simulink model "pi_controllers"  (R2018a)
settings: Solver=VariableStepAuto  StartTime=0.0  StopTime=5  RelTol=1e-3
libraries: fuzblock x1, simulink x1
settings Model: Creator=Iasonas  LastModifiedBy=Iasonas

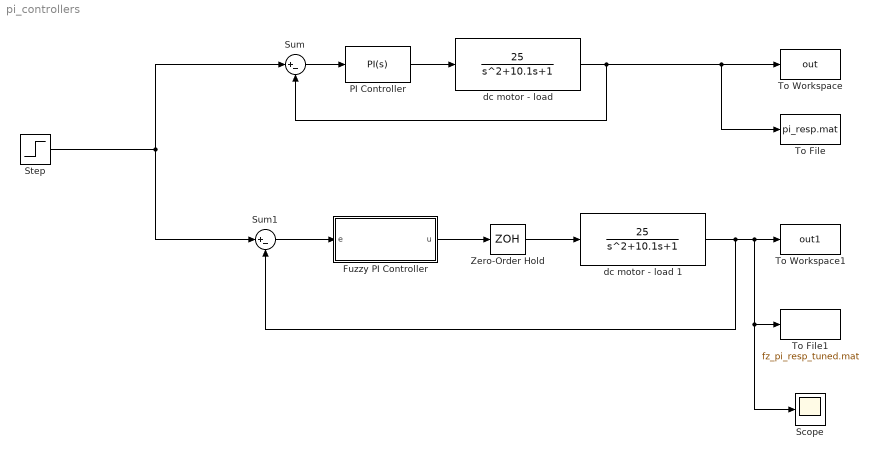
== system pi_controllers ==
  Fuzzy PI Controller : Subsystem
  PI Controller : simulink/Continuous/PID Controller  Controller=PI  TimeDomain=Continuous-time  SampleTime=-1  IntegratorMethod=Forward Euler  FilterMethod=Forward Euler  Form=Parallel  UseFilter=on  ControllerParametersSource=internal  P=2.4  I=0.264  D=0  N=100  InitialConditionSource=internal  InitialConditionForIntegrator=0  InitialConditionForFilter=0  ExternalReset=none  LimitOutput=off  UpperSaturationLimit=inf  LowerSaturationLimit=-inf  LinearizeAsGain=on  AntiWindupMode=none  Kb=1  TrackingMode=off  Kt=1  PParamMin=[]  PParamMax=[]  IParamMin=[]  IParamMax=[]  DParamMin=[]  DParamMax=[]  NParamMin=[]  NParamMax=[]  KbParamMin=[]  KbParamMax=[]  KtParamMin=[]  KtParamMax=[]  POutMin=[]  POutMax=[]  IOutMin=[]  IOutMax=[]  DOutMin=[]  DOutMax=[]  NOutMin=[]  NOutMax=[]  KbOutMin=[]  KbOutMax=[]  KtOutMin=[]  KtOutMax=[]  IntegratorOutMin=[]  IntegratorOutMax=[]  FilterOutMin=[]  FilterOutMax=[]  SumOutMin=[]  SumOutMax=[]  SumI1OutMin=[]  SumI1OutMax=[]  SumI2OutMin=[]  SumI2OutMax=[]  SumI3OutMin=[]  SumI3OutMax=[]  SumDOutMin=[]  SumDOutMax=[]  SaturationOutMin=[]  SaturationOutMax=[]  IntegratorContinuousStateAttributes=''  IntegratorStateMustResolveToSignalObject=off  IntegratorRTWStateStorageClass=Auto  FilterContinuousStateAttributes=''  FilterStateMustResolveToSignalObject=off  FilterRTWStateStorageClass=Auto  DifferentiatorICPrevScaledInput=0  DifferentiatorOutMin=[]  DifferentiatorOutMax=[]  FilterDiffOutCoefMin=[]  FilterDiffOutCoefMax=[]  SumDenOutMin=[]  SumDenOutMax=[]  SumNumOutMin=[]  SumNumOutMax=[]  ReciprocalOutMin=[]  ReciprocalOutMax=[]  DivideOutMin=[]  DivideOutMax=[]  TunerSelectOption=Frequency Response Based
  Scope : Scope
  Step : Step  Time=0.01  After=50  SampleTime=0
  Sum : Sum  Inputs=|+-
  Sum1 : Sum  Inputs=|+-
  To File : ToFile  Filename=pi_resp.mat  MatrixName=resp  SaveFormat=Timeseries
  To File1 : ToFile  Filename=fz_pi_resp_tuned.mat  MatrixName=resp  SaveFormat=Timeseries
  To Workspace : ToWorkspace  VariableName=out  SaveFormat=Timeseries  SampleTime=-1
  To Workspace1 : ToWorkspace  VariableName=out1  SaveFormat=Timeseries  SampleTime=-1
  Zero-Order Hold : ZeroOrderHold  SampleTime=-1
  "dc motor - load " : TransferFcn  Tag=sadsd  Numerator=[25]  Denominator=[1 10.1 1]
      settings: AttributesFormatString=%<RequirementInfo>
  dc motor - load 1 : TransferFcn  Tag=sadsd  Numerator=[25]  Denominator=[1 10.1 1]
      settings: AttributesFormatString=%<RequirementInfo>
  wires:
  PI Controller/1 -> "dc motor - load "/1
  Sum/1 -> PI Controller/1
  "dc motor - load "/1 -> Sum/2, To File/1, To Workspace/1
  Sum1/1 -> Fuzzy PI Controller/1(e)
  dc motor - load 1/1 -> Sum1/2, To File1/1, Scope/1, To Workspace1/1
  Fuzzy PI Controller/1(u) -> Zero-Order Hold/1
  Zero-Order Hold/1 -> dc motor - load 1/1
  Step/1 -> Sum/1, Sum1/1

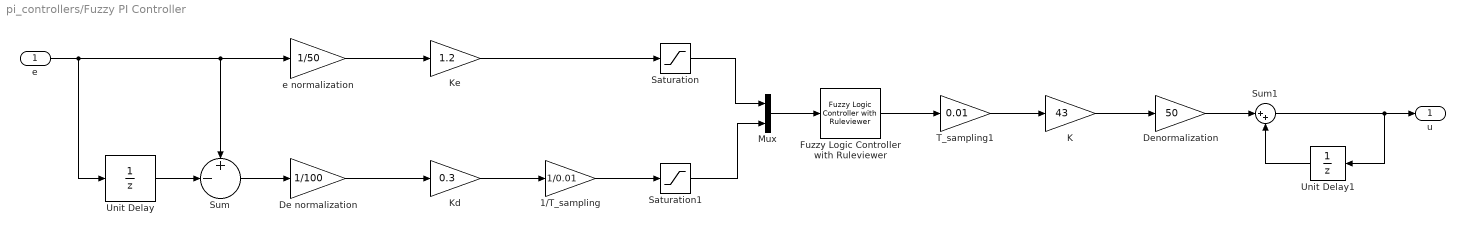
== system pi_controllers/Fuzzy PI Controller ==
  e : Inport
  1/T_sampling : Gain  Gain=1/0.01
  De normalization : Gain  Gain=1/100
  Denormalization : Gain  Gain=50
  Fuzzy Logic Controller with Ruleviewer : fuzblock/Fuzzy Logic  Controller  with Ruleviewer  fismatrix="readfis(\"FZ_PI.fis\")"  Ts=0.022
  Kd : Gain  Gain=0.3
  Ke : Gain  Gain=1.2
  Mux : Mux  Inputs=2
  Saturation : Saturate  UpperLimit=1  LowerLimit=-1
  Saturation1 : Saturate  UpperLimit=1  LowerLimit=-1
  Sum : Sum  Inputs=+-|
  Sum1 : Sum  Inputs=|++
  T_sampling1 : Gain  Gain=0.01
  Unit Delay : UnitDelay  SampleTime=-1
  Unit Delay1 : UnitDelay  SampleTime=-1
  e normalization : Gain  Gain=1/50
  Κ : Gain  Gain=43
  u : Outport
  wires:
  e/1 -> Unit Delay/1, e normalization/1, Sum/1
  Unit Delay/1 -> Sum/2
  Sum/1 -> De normalization/1
  e normalization/1 -> Ke/1
  De normalization/1 -> Kd/1
  Kd/1 -> 1/T_sampling/1
  Ke/1 -> Saturation/1
  1/T_sampling/1 -> Saturation1/1
  Mux/1 -> Fuzzy Logic Controller with Ruleviewer/1
  Saturation/1 -> Mux/1
  Saturation1/1 -> Mux/2
  Fuzzy Logic Controller with Ruleviewer/1 -> T_sampling1/1
  T_sampling1/1 -> Κ/1
  Κ/1 -> Denormalization/1
  Denormalization/1 -> Sum1/1
  Sum1/1 -> Unit Delay1/1, u/1
  Unit Delay1/1 -> Sum1/2
